simulink model "task_2_2c"  (R2021b)
settings: Solver=VariableStepAuto  StartTime=0.0  StopTime=10.0  RelTol=1e-3
libraries: simulink x2
settings Model: Creator=osini  LastModifiedBy=osini

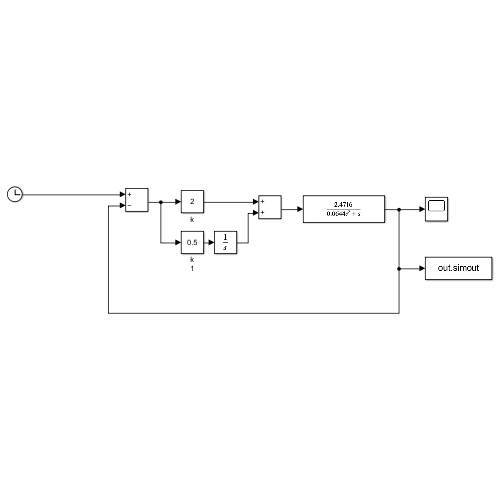
[thumbnail: Simulink's stored preview of the top-level diagram]
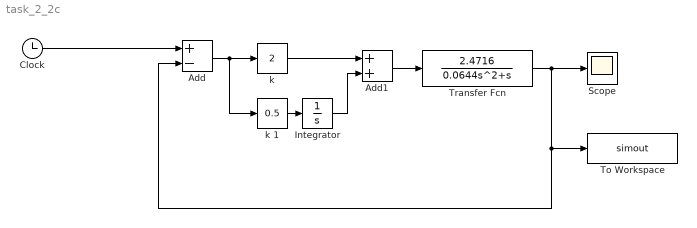
== system task_2_2c ==
  Add : Sum  Inputs=+-
  Add1 : Sum
  Clock : Clock
  Integrator : Integrator
  Scope : Scope
  To Workspace : ToWorkspace  VariableName=simout  SaveFormat=Timeseries  SampleTime=-1
  Transfer Fcn : TransferFcn  Numerator=[2.4716]  Denominator=[0.0644 1 0]
  "k " : simulink/Math Operations/Slider Gain  gain=2  low=0  high=1000
  k 1 : simulink/Math Operations/Slider Gain  gain=0.5  low=0  high=1000
  wires:
  Add/1 -> k 1/1, "k "/1
  Transfer Fcn/1 -> To Workspace/1, Add/2, Scope/1
  Add1/1 -> Transfer Fcn/1
  "k "/1 -> Add1/1
  k 1/1 -> Integrator/1
  Integrator/1 -> Add1/2
  Clock/1 -> Add/1
